simulink model "wlan_phy_tx_pmd"  (Simulink 7.8)
settings: Solver=ode45  StartTime=0.0  StopTime=Sim_Time  RelTol=1e-3
PostLoadFcn:
  | wlan_phy_tx_init
InitFcn:
  | wlan_phy_tx_init
StartFcn:
  | wlan_phy_tx_init
values from neighbouring files (symbols this model uses):
  interleave_64QAM_addr = interleave_64QAM + 2*floor(interleave_64QAM/6)    [wlan_phy_tx_init.m]
  MAX_NUM_BYTES = 4096    [wlan_phy_tx_init.m]
  MAX_NUM_SC = 64    [wlan_phy_tx_init.m]
  Preamble_IQ = PLCP_Preamble.Preamble_t    [wlan_phy_tx_init.m]
  Preamble_IQ_scaled = ALL_MOD_SCALING * Preamble_IQ    [wlan_phy_tx_init.m]
  Sim_Tx_Start_Period = 1*(160 * Tx_Time_usec) + 2e3    [wlan_phy_tx_init.m]
undefined symbols (not defined in the file or in its folder): gcbh, interleave_16QAM, interleave_bpsk, interleave_QPSK, Mod_Constellation_16QAM, Mod_Constellation_64QAM, Mod_Constellation_BPSK, Mod_Constellation_QPSK, xlBlockLoadCallback, xlGetNormalizedPeriod
libraries: xbsIndex_r4 x1173, xbsEDKLib_r4 x1
(part 5 of 8)

== system wlan_phy_tx_pmd/FIFO/I/Q Slice ==
  IQ : Inport
  Reinterpret2 : xbsIndex_r4/Reinterpret  force_arith_type=on  arith_type="Signed  (2's comp)"  force_bin_pt=on  bin_pt=15  block_type=reinterpret
  Reinterpret3 : xbsIndex_r4/Reinterpret  force_arith_type=on  arith_type="Signed  (2's comp)"  force_bin_pt=on  bin_pt=15  block_type=reinterpret
  Slice : xbsIndex_r4/Slice  nbits=16  boolean_output=off  mode=Upper Bit Location + Width  bit1=0  base1=MSB of Input  bit0=0  base0=LSB of Input  dbl_ovrd=off  block_type=slice
  Slice1 : xbsIndex_r4/Slice  nbits=16  boolean_output=off  mode=Lower Bit Location + Width  bit1=0  base1=MSB of Input  bit0=0  base0=LSB of Input  dbl_ovrd=off  block_type=slice
  I : Outport
  Q : Outport  Port=2
  wires:
  Reinterpret3/1 -> Q/1
  Reinterpret2/1 -> I/1
  IQ/1 -> Slice/1, Slice1/1
  Slice1/1 -> Reinterpret3/1
  Slice/1 -> Reinterpret2/1

== system wlan_phy_tx_pmd/Interleave & Modulate/16-QAM ==
  New Sym : Inport
  "bit tdata " : Inport  Port=2
  "bit tvalid " : Inport  Port=3
  data sym addr : Inport  Port=4
  16QAM Int Addr : Subsystem
  "16QAM Intlv " : Scope  NumInputPorts=7
      settings: TimeRange=15000  YMin=0~0~0~-0.1~0~0~-1  YMax=1~250~1~1.1~120~3~1  SaveName=ScopeData23
  Bit Memory1 : xbsIndex_r4/Dual Port RAM  depth=512  initVector=0  distributed_mem=Block RAM  init_a=0  init_b=0  rst_a=off  rst_b=off  en_a=off  en_b=off  latency=1  write_mode_A=Read After Write  write_mode_B=Read After Write  dbl_ovrd=off  optimize=Area  block_type=dpram
  Concat1 : xbsIndex_r4/Concat  num_inputs=2  dbl_ovrd=off  block_type=concat
  Concat2 : xbsIndex_r4/Concat  num_inputs=2  dbl_ovrd=off  block_type=concat
  Constant1 : xbsIndex_r4/Constant  const=0  gui_display_data_type=Fixed-point  arith_type=Unsigned  n_bits=4  bin_pt=0  preci_type=Single  exp_width=8  frac_width=24  explicit_period=off  period=1  equ=P=C  opselect=C  inp2=PCIN>>17  opr=+  inp1=P  carry=CIN  dbl_ovrd=off  block_type=constant
  Constant2 : xbsIndex_r4/Constant  const=0  gui_display_data_type=Boolean  arith_type=Boolean  n_bits=1  bin_pt=0  preci_type=Single  exp_width=8  frac_width=24  explicit_period=off  period=1  equ=P=C  opselect=C  inp2=PCIN>>17  opr=+  inp1=P  carry=CIN  dbl_ovrd=off  block_type=constant
  Delay2 : xbsIndex_r4/Delay  rst=off  infoeditControl=Selection of Reset will increase slice count due to use of real FFs and instead of SRLs  en=off  latency=1  dbl_ovrd=off  reg_retiming=off  block_type=delay
  Delay6 : xbsIndex_r4/Delay  rst=off  infoeditControl=Selection of Reset will increase slice count due to use of real FFs and instead of SRLs  en=off  latency=1  dbl_ovrd=off  reg_retiming=off  block_type=delay
  Gateway Out{1..5,8} (6 alike) : xbsIndex_r4/Gateway Out  inherit_from_input=off  hdl_port=off  timing_constraint=None  locs_specified=off  LOCs={}  UseAsDAC=off  DACChannel='1'  block_type=gatewayout
  Inverter : xbsIndex_r4/Inverter  en=off  latency=0  dbl_ovrd=off  block_type=inv
  Terminator : Terminator
  4b Data : Outport
  wires:
  Bit Memory1/2 -> 4b Data/1, Gateway Out5/1
  Bit Memory1/1 -> Terminator/1
  Inverter/1 -> Concat2/1
  data sym addr/1 -> Concat2/2
  Concat2/1 -> Bit Memory1/4, Gateway Out4/1
  Concat1/1 -> Bit Memory1/1, Gateway Out1/1
  16QAM Int Addr/2(Wr Addr) -> Concat1/2
  16QAM Int Addr/1(Wr Offset) -> Inverter/1, Concat1/1
  "bit tdata "/1 -> Delay6/1
  Constant2/1 -> Bit Memory1/6
  Constant1/1 -> Bit Memory1/5
  New Sym/1 -> 16QAM Int Addr/1(New Sym), Gateway Out8/1
  "bit tvalid "/1 -> 16QAM Int Addr/2(Bit Valid), Delay2/1
  Delay6/1 -> Bit Memory1/2, Gateway Out2/1
  Delay2/1 -> Bit Memory1/3, Gateway Out3/1
  Gateway Out8/1 -> "16QAM Intlv "/1  "New Sym"
  Gateway Out1/1 -> "16QAM Intlv "/2  "Wr Addr"
  Gateway Out2/1 -> "16QAM Intlv "/3  "Wr Bit"
  Gateway Out3/1 -> "16QAM Intlv "/4  "Wr En"
  Gateway Out4/1 -> "16QAM Intlv "/5  "Rd Addr"
  Gateway Out5/1 -> "16QAM Intlv "/6  "Rd Sym Out"

== system wlan_phy_tx_pmd/Interleave & Modulate/16QAM Mod ==
  note: 16-QAM Bit Mapping:
      | [b0 b1] / [b2 b3]:
      | 00 = -3
      | 01 = -1
      | 11 = +1
      | 10 = +3
      | Norm = 1/sqrt(10)
  note: 00 -> 00
  note: 10 -> 01
  note: 01 -> 10
  note: 11 -> 11
  b[3:0] : Inport
  Constant1 : xbsIndex_r4/Constant  const=Mod_Constellation_16QAM(3)  gui_display_data_type=Fixed-point  arith_type=Signed (2's comp)  n_bits=12  bin_pt=11  preci_type=Single  exp_width=8  frac_width=24  explicit_period=off  period=1  equ=P=C  opselect=C  inp2=PCIN>>17  opr=+  inp1=P  carry=CIN  dbl_ovrd=off  block_type=constant
  Constant2 : xbsIndex_r4/Constant  const=Mod_Constellation_16QAM(1)  gui_display_data_type=Fixed-point  arith_type=Signed (2's comp)  n_bits=12  bin_pt=11  preci_type=Single  exp_width=8  frac_width=24  explicit_period=off  period=1  equ=P=C  opselect=C  inp2=PCIN>>17  opr=+  inp1=P  carry=CIN  dbl_ovrd=off  block_type=constant
  Constant3 : xbsIndex_r4/Constant  const=Mod_Constellation_16QAM(2)  gui_display_data_type=Fixed-point  arith_type=Signed (2's comp)  n_bits=12  bin_pt=11  preci_type=Single  exp_width=8  frac_width=24  explicit_period=off  period=1  equ=P=C  opselect=C  inp2=PCIN>>17  opr=+  inp1=P  carry=CIN  dbl_ovrd=off  block_type=constant
  Constant4 : xbsIndex_r4/Constant  const=Mod_Constellation_16QAM(4)  gui_display_data_type=Fixed-point  arith_type=Signed (2's comp)  n_bits=12  bin_pt=11  preci_type=Single  exp_width=8  frac_width=24  explicit_period=off  period=1  equ=P=C  opselect=C  inp2=PCIN>>17  opr=+  inp1=P  carry=CIN  dbl_ovrd=off  block_type=constant
  Mux : xbsIndex_r4/Mux  inputs=4  en=off  latency=0  precision=Full  arith_type=Unsigned  n_bits=16  bin_pt=14  quantization=Truncate  overflow=Wrap  dbl_ovrd=off  block_type=mux
  Mux1 : xbsIndex_r4/Mux  inputs=4  en=off  latency=0  precision=Full  arith_type=Unsigned  n_bits=16  bin_pt=14  quantization=Truncate  overflow=Wrap  dbl_ovrd=off  block_type=mux
  b[1:0] : xbsIndex_r4/Slice  nbits=2  boolean_output=off  mode=Lower Bit Location + Width  bit1=0  base1=MSB of Input  bit0=0  base0=LSB of Input  dbl_ovrd=off  block_type=slice
  b[3:2] : xbsIndex_r4/Slice  nbits=2  boolean_output=off  mode=Lower Bit Location + Width  bit1=0  base1=MSB of Input  bit0=2  base0=LSB of Input  dbl_ovrd=off  block_type=slice
  I : Outport
  Q : Outport  Port=2
  wires:
  b[1:0]/1 -> Mux/1
  b[3:0]/1 -> b[1:0]/1, b[3:2]/1
  Constant2/1 -> Mux/2, Mux1/2
  Constant1/1 -> Mux/3, Mux1/3
  Constant3/1 -> Mux/4, Mux1/4
  Constant4/1 -> Mux/5, Mux1/5
  b[3:2]/1 -> Mux1/1
  Mux/1 -> I/1
  Mux1/1 -> Q/1

== system wlan_phy_tx_pmd/Interleave & Modulate/64-QAM ==
  New Sym : Inport
  "bit tdata " : Inport  Port=2
  "bit tvalid " : Inport  Port=3
  data sym addr : Inport  Port=4
  64QAM Int Addr : Subsystem
  "64QAM Intlv " : Scope  NumInputPorts=7
      settings: TimeRange=10000  YMin=0~0~0~-0.1~0~0~-1  YMax=1~250~1~1.1~120~3~1  SaveName=ScopeData23
  Bit Memory1 : xbsIndex_r4/Dual Port RAM  depth=1024  initVector=0  distributed_mem=Block RAM  init_a=0  init_b=0  rst_a=off  rst_b=off  en_a=off  en_b=off  latency=1  write_mode_A=Read After Write  write_mode_B=Read After Write  dbl_ovrd=off  optimize=Area  block_type=dpram
  Concat1 : xbsIndex_r4/Concat  num_inputs=2  dbl_ovrd=off  block_type=concat
  Concat2 : xbsIndex_r4/Concat  num_inputs=2  dbl_ovrd=off  block_type=concat
  Constant1 : xbsIndex_r4/Constant  const=0  gui_display_data_type=Fixed-point  arith_type=Unsigned  n_bits=8  bin_pt=0  preci_type=Single  exp_width=8  frac_width=24  explicit_period=off  period=1  equ=P=C  opselect=C  inp2=PCIN>>17  opr=+  inp1=P  carry=CIN  dbl_ovrd=off  block_type=constant
  Constant2 : xbsIndex_r4/Constant  const=0  gui_display_data_type=Boolean  arith_type=Boolean  n_bits=1  bin_pt=0  preci_type=Single  exp_width=8  frac_width=24  explicit_period=off  period=1  equ=P=C  opselect=C  inp2=PCIN>>17  opr=+  inp1=P  carry=CIN  dbl_ovrd=off  block_type=constant
  Delay2 : xbsIndex_r4/Delay  rst=off  infoeditControl=Selection of Reset will increase slice count due to use of real FFs and instead of SRLs  en=off  latency=1  dbl_ovrd=off  reg_retiming=off  block_type=delay
  Delay6 : xbsIndex_r4/Delay  rst=off  infoeditControl=Selection of Reset will increase slice count due to use of real FFs and instead of SRLs  en=off  latency=1  dbl_ovrd=off  reg_retiming=off  block_type=delay
  Gateway Out{1..6,8} (7 alike) : xbsIndex_r4/Gateway Out  inherit_from_input=off  hdl_port=off  timing_constraint=None  locs_specified=off  LOCs={}  UseAsDAC=off  DACChannel='1'  block_type=gatewayout
  Inverter : xbsIndex_r4/Inverter  en=off  latency=0  dbl_ovrd=off  block_type=inv
  Slice : xbsIndex_r4/Slice  nbits=6  boolean_output=off  mode=Lower Bit Location + Width  bit1=0  base1=MSB of Input  bit0=0  base0=LSB of Input  dbl_ovrd=off  block_type=slice
  Terminator : Terminator
  6b Data : Outport
  wires:
  Gateway Out5/1 -> "64QAM Intlv "/6  "Rd Sym Out"
  Gateway Out4/1 -> "64QAM Intlv "/5  "Rd Addr"
  Gateway Out3/1 -> "64QAM Intlv "/4  "Wr En"
  Gateway Out2/1 -> "64QAM Intlv "/3  "Wr Bit"
  Gateway Out1/1 -> "64QAM Intlv "/2  "Wr Addr"
  Gateway Out8/1 -> "64QAM Intlv "/1  "New Sym"
  Delay2/1 -> Gateway Out3/1, Bit Memory1/3
  Delay6/1 -> Gateway Out2/1, Bit Memory1/2
  "bit tvalid "/1 -> Delay2/1, 64QAM Int Addr/2(Bit Valid)
  New Sym/1 -> Gateway Out8/1, 64QAM Int Addr/1(New Sym)
  Constant1/1 -> Bit Memory1/5
  Constant2/1 -> Bit Memory1/6
  "bit tdata "/1 -> Delay6/1
  64QAM Int Addr/1(Wr Offset) -> Concat1/1, Inverter/1
  64QAM Int Addr/2(Wr Addr) -> Concat1/2
  Concat1/1 -> Gateway Out1/1, Bit Memory1/1
  Concat2/1 -> Gateway Out4/1, Bit Memory1/4
  data sym addr/1 -> Concat2/2
  Inverter/1 -> Concat2/1
  Bit Memory1/1 -> Terminator/1
  Bit Memory1/2 -> Gateway Out5/1, Slice/1
  Slice/1 -> 6b Data/1, Gateway Out6/1
  Gateway Out6/1 -> "64QAM Intlv "/7

== system wlan_phy_tx_pmd/Interleave & Modulate/64QAM Mod ==
  note: 64-QAM Bit Mapping:
      | [b0 b1 b2] / [b3 b4 b5]:
      | 000 = -7
      | 001 = -5
      | 010 = -1
      | 011 = -3
      | 100 = +7
      | 101 = +5
      | 110 = +1
      | 111 = +3
      |
      | Norm = 1/sqrt(42)
  note: Endian swap here - mux sel is [b2 b1 b0] / [b5 b4 b3]
  note: 000
  note: 001
  note: 010
  note: 011
  note: 100
  note: 101
  note: 110
  note: 111
  b[5:0] : Inport
  Constant1 : xbsIndex_r4/Constant  const=Mod_Constellation_64QAM(5)  gui_display_data_type=Fixed-point  arith_type=Signed (2's comp)  n_bits=12  bin_pt=11  preci_type=Single  exp_width=8  frac_width=24  explicit_period=off  period=1  equ=P=C  opselect=C  inp2=PCIN>>17  opr=+  inp1=P  carry=CIN  dbl_ovrd=off  block_type=constant
  Constant10 : xbsIndex_r4/Constant  const=Mod_Constellation_64QAM(2)  gui_display_data_type=Fixed-point  arith_type=Signed (2's comp)  n_bits=12  bin_pt=11  preci_type=Single  exp_width=8  frac_width=24  explicit_period=off  period=1  equ=P=C  opselect=C  inp2=PCIN>>17  opr=+  inp1=P  carry=CIN  dbl_ovrd=off  block_type=constant
  Constant11 : xbsIndex_r4/Constant  const=Mod_Constellation_64QAM(4)  gui_display_data_type=Fixed-point  arith_type=Signed (2's comp)  n_bits=12  bin_pt=11  preci_type=Single  exp_width=8  frac_width=24  explicit_period=off  period=1  equ=P=C  opselect=C  inp2=PCIN>>17  opr=+  inp1=P  carry=CIN  dbl_ovrd=off  block_type=constant
  Constant12 : xbsIndex_r4/Constant  const=Mod_Constellation_64QAM(8)  gui_display_data_type=Fixed-point  arith_type=Signed (2's comp)  n_bits=12  bin_pt=11  preci_type=Single  exp_width=8  frac_width=24  explicit_period=off  period=1  equ=P=C  opselect=C  inp2=PCIN>>17  opr=+  inp1=P  carry=CIN  dbl_ovrd=off  block_type=constant
  Constant13 : xbsIndex_r4/Constant  const=Mod_Constellation_64QAM(1)  gui_display_data_type=Fixed-point  arith_type=Signed (2's comp)  n_bits=12  bin_pt=11  preci_type=Single  exp_width=8  frac_width=24  explicit_period=off  period=1  equ=P=C  opselect=C  inp2=PCIN>>17  opr=+  inp1=P  carry=CIN  dbl_ovrd=off  block_type=constant
  Constant14 : xbsIndex_r4/Constant  const=Mod_Constellation_64QAM(3)  gui_display_data_type=Fixed-point  arith_type=Signed (2's comp)  n_bits=12  bin_pt=11  preci_type=Single  exp_width=8  frac_width=24  explicit_period=off  period=1  equ=P=C  opselect=C  inp2=PCIN>>17  opr=+  inp1=P  carry=CIN  dbl_ovrd=off  block_type=constant
  Constant15 : xbsIndex_r4/Constant  const=Mod_Constellation_64QAM(7)  gui_display_data_type=Fixed-point  arith_type=Signed (2's comp)  n_bits=12  bin_pt=11  preci_type=Single  exp_width=8  frac_width=24  explicit_period=off  period=1  equ=P=C  opselect=C  inp2=PCIN>>17  opr=+  inp1=P  carry=CIN  dbl_ovrd=off  block_type=constant
  Constant16 : xbsIndex_r4/Constant  const=Mod_Constellation_64QAM(6)  gui_display_data_type=Fixed-point  arith_type=Signed (2's comp)  n_bits=12  bin_pt=11  preci_type=Single  exp_width=8  frac_width=24  explicit_period=off  period=1  equ=P=C  opselect=C  inp2=PCIN>>17  opr=+  inp1=P  carry=CIN  dbl_ovrd=off  block_type=constant
  Constant2 : xbsIndex_r4/Constant  const=Mod_Constellation_64QAM(1)  gui_display_data_type=Fixed-point  arith_type=Signed (2's comp)  n_bits=12  bin_pt=11  preci_type=Single  exp_width=8  frac_width=24  explicit_period=off  period=1  equ=P=C  opselect=C  inp2=PCIN>>17  opr=+  inp1=P  carry=CIN  dbl_ovrd=off  block_type=constant
  Constant3 : xbsIndex_r4/Constant  const=Mod_Constellation_64QAM(3)  gui_display_data_type=Fixed-point  arith_type=Signed (2's comp)  n_bits=12  bin_pt=11  preci_type=Single  exp_width=8  frac_width=24  explicit_period=off  period=1  equ=P=C  opselect=C  inp2=PCIN>>17  opr=+  inp1=P  carry=CIN  dbl_ovrd=off  block_type=constant
  Constant4 : xbsIndex_r4/Constant  const=Mod_Constellation_64QAM(7)  gui_display_data_type=Fixed-point  arith_type=Signed (2's comp)  n_bits=12  bin_pt=11  preci_type=Single  exp_width=8  frac_width=24  explicit_period=off  period=1  equ=P=C  opselect=C  inp2=PCIN>>17  opr=+  inp1=P  carry=CIN  dbl_ovrd=off  block_type=constant
  Constant5 : xbsIndex_r4/Constant  const=Mod_Constellation_64QAM(5)  gui_display_data_type=Fixed-point  arith_type=Signed (2's comp)  n_bits=12  bin_pt=11  preci_type=Single  exp_width=8  frac_width=24  explicit_period=off  period=1  equ=P=C  opselect=C  inp2=PCIN>>17  opr=+  inp1=P  carry=CIN  dbl_ovrd=off  block_type=constant
  Constant6 : xbsIndex_r4/Constant  const=Mod_Constellation_64QAM(2)  gui_display_data_type=Fixed-point  arith_type=Signed (2's comp)  n_bits=12  bin_pt=11  preci_type=Single  exp_width=8  frac_width=24  explicit_period=off  period=1  equ=P=C  opselect=C  inp2=PCIN>>17  opr=+  inp1=P  carry=CIN  dbl_ovrd=off  block_type=constant
  Constant7 : xbsIndex_r4/Constant  const=Mod_Constellation_64QAM(4)  gui_display_data_type=Fixed-point  arith_type=Signed (2's comp)  n_bits=12  bin_pt=11  preci_type=Single  exp_width=8  frac_width=24  explicit_period=off  period=1  equ=P=C  opselect=C  inp2=PCIN>>17  opr=+  inp1=P  carry=CIN  dbl_ovrd=off  block_type=constant
  Constant8 : xbsIndex_r4/Constant  const=Mod_Constellation_64QAM(8)  gui_display_data_type=Fixed-point  arith_type=Signed (2's comp)  n_bits=12  bin_pt=11  preci_type=Single  exp_width=8  frac_width=24  explicit_period=off  period=1  equ=P=C  opselect=C  inp2=PCIN>>17  opr=+  inp1=P  carry=CIN  dbl_ovrd=off  block_type=constant
  Constant9 : xbsIndex_r4/Constant  const=Mod_Constellation_64QAM(6)  gui_display_data_type=Fixed-point  arith_type=Signed (2's comp)  n_bits=12  bin_pt=11  preci_type=Single  exp_width=8  frac_width=24  explicit_period=off  period=1  equ=P=C  opselect=C  inp2=PCIN>>17  opr=+  inp1=P  carry=CIN  dbl_ovrd=off  block_type=constant
  Mux : xbsIndex_r4/Mux  inputs=8  en=off  latency=0  precision=Full  arith_type=Unsigned  n_bits=16  bin_pt=14  quantization=Truncate  overflow=Wrap  dbl_ovrd=off  block_type=mux
  Mux1 : xbsIndex_r4/Mux  inputs=8  en=off  latency=0  precision=Full  arith_type=Unsigned  n_bits=16  bin_pt=14  quantization=Truncate  overflow=Wrap  dbl_ovrd=off  block_type=mux
  b[2:0] : xbsIndex_r4/Slice  nbits=3  boolean_output=off  mode=Lower Bit Location + Width  bit1=0  base1=MSB of Input  bit0=0  base0=LSB of Input  dbl_ovrd=off  block_type=slice
  b[5:3] : xbsIndex_r4/Slice  nbits=3  boolean_output=off  mode=Lower Bit Location + Width  bit1=0  base1=MSB of Input  bit0=3  base0=LSB of Input  dbl_ovrd=off  block_type=slice
  I : Outport
  Q : Outport  Port=2
  wires:
  Constant4/1 -> Mux/5
  Constant3/1 -> Mux/4
  Constant1/1 -> Mux/3
  Constant2/1 -> Mux/2
  b[5:0]/1 -> b[5:3]/1, b[2:0]/1
  b[2:0]/1 -> Mux/1
  Constant10/1 -> Mux/6
  Constant9/1 -> Mux/7
  Constant11/1 -> Mux/8
  Constant12/1 -> Mux/9
  Mux/1 -> I/1
  Constant15/1 -> Mux1/5
  Constant14/1 -> Mux1/4
  Constant5/1 -> Mux1/3
  Constant13/1 -> Mux1/2
  Constant6/1 -> Mux1/6
  Constant16/1 -> Mux1/7
  Constant7/1 -> Mux1/8
  Constant8/1 -> Mux1/9
  b[5:3]/1 -> Mux1/1
  Mux1/1 -> Q/1

== system wlan_phy_tx_pmd/Interleave & Modulate/BPSK ==
  New Sym : Inport
  "bit tdata " : Inport  Port=2
  "bit tvalid " : Inport  Port=3
  data sym addr : Inport  Port=4
  BPSK Int Addr : Subsystem
  "BSPK Intlv " : Scope  NumInputPorts=7
      settings: TimeRange=10000  YMin=0~0~-0.1~-2~0~-0.1~-0.1  YMax=300~300~1.1~2~4000~1.1~1.1  SaveName=ScopeData15
  Bit Memory : xbsIndex_r4/Dual Port RAM  depth=128  initVector=0  distributed_mem=Block RAM  init_a=0  init_b=0  rst_a=off  rst_b=off  en_a=off  en_b=off  latency=1  write_mode_A=Read After Write  write_mode_B=Read After Write  dbl_ovrd=off  optimize=Area  block_type=dpram
  Concat1 : xbsIndex_r4/Concat  num_inputs=2  dbl_ovrd=off  block_type=concat
  Concat2 : xbsIndex_r4/Concat  num_inputs=2  dbl_ovrd=off  block_type=concat
  Constant1 : xbsIndex_r4/Constant  const=0  gui_display_data_type=Fixed-point  arith_type=Unsigned  n_bits=1  bin_pt=0  preci_type=Single  exp_width=8  frac_width=24  explicit_period=off  period=1  equ=P=C  opselect=C  inp2=PCIN>>17  opr=+  inp1=P  carry=CIN  dbl_ovrd=off  block_type=constant
  Constant2 : xbsIndex_r4/Constant  const=0  gui_display_data_type=Boolean  arith_type=Boolean  n_bits=1  bin_pt=0  preci_type=Single  exp_width=8  frac_width=24  explicit_period=off  period=1  equ=P=C  opselect=C  inp2=PCIN>>17  opr=+  inp1=P  carry=CIN  dbl_ovrd=off  block_type=constant
  Delay1 : xbsIndex_r4/Delay  rst=off  infoeditControl=Selection of Reset will increase slice count due to use of real FFs and instead of SRLs  en=off  latency=1  dbl_ovrd=off  reg_retiming=off  block_type=delay
  Delay6 : xbsIndex_r4/Delay  rst=off  infoeditControl=Selection of Reset will increase slice count due to use of real FFs and instead of SRLs  en=off  latency=1  dbl_ovrd=off  reg_retiming=off  block_type=delay
  Gateway Out{1..5,8} (6 alike) : xbsIndex_r4/Gateway Out  inherit_from_input=off  hdl_port=off  timing_constraint=None  locs_specified=off  LOCs={}  UseAsDAC=off  DACChannel='1'  block_type=gatewayout
  Inverter : xbsIndex_r4/Inverter  en=off  latency=0  dbl_ovrd=off  block_type=inv
  Terminator : Terminator
  1b Data : Outport
  wires:
  "bit tvalid "/1 -> BPSK Int Addr/2(Bit Valid), Delay1/1
  New Sym/1 -> BPSK Int Addr/1(New Sym), Gateway Out8/1
  Constant1/1 -> Bit Memory/5
  Constant2/1 -> Bit Memory/6
  "bit tdata "/1 -> Delay6/1
  BPSK Int Addr/1(Wr Offset) -> Concat1/1, Inverter/1
  BPSK Int Addr/2(Wr Addr) -> Concat1/2
  Concat1/1 -> Bit Memory/1, Gateway Out1/1
  Concat2/1 -> Bit Memory/4, Gateway Out4/1
  data sym addr/1 -> Concat2/2
  Inverter/1 -> Concat2/1
  Bit Memory/1 -> Terminator/1
  Bit Memory/2 -> 1b Data/1, Gateway Out5/1
  Gateway Out8/1 -> "BSPK Intlv "/1
  Gateway Out1/1 -> "BSPK Intlv "/2
  Gateway Out2/1 -> "BSPK Intlv "/3
  Gateway Out3/1 -> "BSPK Intlv "/4
  Gateway Out4/1 -> "BSPK Intlv "/5
  Gateway Out5/1 -> "BSPK Intlv "/6
  Delay6/1 -> Bit Memory/2, Gateway Out2/1
  Delay1/1 -> Bit Memory/3, Gateway Out3/1

== system wlan_phy_tx_pmd/Interleave & Modulate/BPSK Mod ==
  b[0] : Inport
  Constant2 : xbsIndex_r4/Constant  const=Mod_Constellation_BPSK(1)  gui_display_data_type=Fixed-point  arith_type=Signed (2's comp)  n_bits=12  bin_pt=11  preci_type=Single  exp_width=8  frac_width=24  explicit_period=off  period=1  equ=P=C  opselect=C  inp2=PCIN>>17  opr=+  inp1=P  carry=CIN  dbl_ovrd=off  block_type=constant
  Constant3 : xbsIndex_r4/Constant  const=Mod_Constellation_BPSK(2)  gui_display_data_type=Fixed-point  arith_type=Signed (2's comp)  n_bits=12  bin_pt=11  preci_type=Single  exp_width=8  frac_width=24  explicit_period=off  period=1  equ=P=C  opselect=C  inp2=PCIN>>17  opr=+  inp1=P  carry=CIN  dbl_ovrd=off  block_type=constant
  Constant4 : xbsIndex_r4/Constant  const=0  gui_display_data_type=Fixed-point  arith_type=Signed (2's comp)  n_bits=12  bin_pt=11  preci_type=Single  exp_width=8  frac_width=24  explicit_period=off  period=1  equ=P=C  opselect=C  inp2=PCIN>>17  opr=+  inp1=P  carry=CIN  dbl_ovrd=off  block_type=constant
  Mux : xbsIndex_r4/Mux  inputs=2  en=off  latency=0  precision=Full  arith_type=Unsigned  n_bits=16  bin_pt=14  quantization=Truncate  overflow=Wrap  dbl_ovrd=off  block_type=mux
  I : Outport
  Q : Outport  Port=2
  wires:
  Mux/1 -> I/1
  Constant3/1 -> Mux/3
  Constant2/1 -> Mux/2
  b[0]/1 -> Mux/1
  Constant4/1 -> Q/1

== system wlan_phy_tx_pmd/Interleave & Modulate/Coded Bit Counter ==
  Bit valid : Inport
  Constant3 : xbsIndex_r4/Constant  const=48  gui_display_data_type=Fixed-point  arith_type=Unsigned  n_bits=6  bin_pt=0  preci_type=Single  exp_width=8  frac_width=24  explicit_period=off  period=1  equ=P=C  opselect=C  inp2=PCIN>>17  opr=+  inp1=P  carry=CIN  dbl_ovrd=off  block_type=constant
  Delay2 : xbsIndex_r4/Delay  rst=off  infoeditControl=Selection of Reset will increase slice count due to use of real FFs and instead of SRLs  en=off  latency=1  dbl_ovrd=off  reg_retiming=off  block_type=delay
  Gateway Out{1..4,8} (5 alike) : xbsIndex_r4/Gateway Out  inherit_from_input=off  hdl_port=off  timing_constraint=None  locs_specified=off  LOCs={}  UseAsDAC=off  DACChannel='1'  block_type=gatewayout
  Inverter : xbsIndex_r4/Inverter  en=off  latency=0  dbl_ovrd=off  block_type=inv
      settings: xl_area=[0 0 0 0 0 0 0]  block_version=VER_STRING_GOES_HERE
  Logical1 : xbsIndex_r4/Logical  logical_function=OR  inputs=2  en=off  latency=0  precision=Full  arith_type=Unsigned  n_bits=8  bin_pt=2  align_bp=on  dbl_ovrd=off  block_type=logical
      settings: xl_area=[1 0 0 1 0 0 0]  block_version=VER_STRING_GOES_HERE
  Logical2 : xbsIndex_r4/Logical  logical_function=AND  inputs=2  en=off  latency=0  precision=Full  arith_type=Unsigned  n_bits=8  bin_pt=2  align_bp=on  dbl_ovrd=off  block_type=logical
      settings: xl_area=[1 0 0 1 0 0 0]  block_version=VER_STRING_GOES_HERE
  Mux : xbsIndex_r4/Mux  inputs=2  en=off  latency=0  precision=Full  arith_type=Unsigned  n_bits=16  bin_pt=14  quantization=Truncate  overflow=Wrap  dbl_ovrd=off  block_type=mux
  Relational2 : xbsIndex_r4/Relational  mode=a<b  en=off  latency=0  dbl_ovrd=off  block_type=relational
  S-R Latch2 : Subsystem
  Sym Coded Bit Count : xbsIndex_r4/Counter  cnt_type=Free Running  cnt_to=Inf  operation=Up  start_count=1  cnt_by_val=1  arith_type=Unsigned  n_bits=9  bin_pt=0  load_pin=off  rst=on  en=on  explicit_period=off  period=1  dbl_ovrd=off  use_behavioral_HDL=off  implementation=Fabric  block_type=counter
  Sym Coded Bit Count1 : Scope  NumInputPorts=7
      settings: TimeRange=15000  YMin=0~0~0~0~0~-1~-1  YMax=1~100~1~1~1~1~1  SaveName=ScopeData5
  Bits Ready : Outport
  wires:
  [DATA_N_CBPS] -> Mux/3
  Constant3/1 -> Mux/2
  Mux/1 -> Relational2/2
  Sym Coded Bit Count/1 -> Gateway Out1/1, Relational2/1
  Logical1/1 -> Sym Coded Bit Count/1
  S-R Latch2/1(Q) -> Mux/1, Gateway Out4/1
  Bit valid/1 -> Sym Coded Bit Count/2, Gateway Out8/1, Logical2/2
  Logical2/1 -> Logical1/1, S-R Latch2/1(S), Gateway Out3/1, Delay2/1
  [TX_RESET] -> S-R Latch2/2(R), Logical1/2
  Gateway Out8/1 -> Sym Coded Bit Count1/1
  Gateway Out1/1 -> Sym Coded Bit Count1/2
  Gateway Out2/1 -> Sym Coded Bit Count1/3
  Gateway Out3/1 -> Sym Coded Bit Count1/4
  Gateway Out4/1 -> Sym Coded Bit Count1/5
  Delay2/1 -> Bits Ready/1
  Relational2/1 -> Inverter/1
  Inverter/1 -> Logical2/1, Gateway Out2/1

== system wlan_phy_tx_pmd/Interleave & Modulate/Control & Pilots ==
  note: SC Counter EN high extra cycle post wrap reset
      | (due to SR latch latency?)
  note: 1 cycle for RAM access
  note: May need tweaked delay to handle edge
      | case of 1 required bit alone in final
      | symbol
  Bits Ready : Inport
  FIFO Ready : Inport  Port=2
  Concat1 : xbsIndex_r4/Concat  num_inputs=2  dbl_ovrd=off  block_type=concat
  Data SC Map : Subsystem
  Delay{,1..3,5..6} (6 alike) : xbsIndex_r4/Delay  rst=off  infoeditControl=Selection of Reset will increase slice count due to use of real FFs and instead of SRLs  en=off  latency=1  dbl_ovrd=off  reg_retiming=off  block_type=delay
  Delay4 : xbsIndex_r4/Delay  rst=off  infoeditControl=Selection of Reset will increase slice count due to use of real FFs and instead of SRLs  en=off  latency=0  dbl_ovrd=off  reg_retiming=off  block_type=delay
  Gateway Out{1..4,8} (5 alike) : xbsIndex_r4/Gateway Out  inherit_from_input=off  hdl_port=off  timing_constraint=None  locs_specified=off  LOCs={}  UseAsDAC=off  DACChannel='1'  block_type=gatewayout
  Logical : xbsIndex_r4/Logical  logical_function=OR  inputs=2  en=off  latency=0  precision=Full  arith_type=Unsigned  n_bits=8  bin_pt=2  align_bp=on  dbl_ovrd=off  block_type=logical
      settings: xl_area=[0, 0, 0, 0, 0, 0, 0]  block_version=VER_STRING_GOES_HERE
  Logical1 : xbsIndex_r4/Logical  logical_function=AND  inputs=2  en=off  latency=0  precision=Full  arith_type=Unsigned  n_bits=8  bin_pt=2  align_bp=on  dbl_ovrd=off  block_type=logical
      settings: xl_area=[0, 0, 0, 0, 0, 0, 0]  block_version=VER_STRING_GOES_HERE
  Logical2 : xbsIndex_r4/Logical  logical_function=AND  inputs=2  en=off  latency=0  precision=Full  arith_type=Unsigned  n_bits=8  bin_pt=2  align_bp=on  dbl_ovrd=off  block_type=logical
      settings: xl_area=[0, 0, 0, 0, 0, 0, 0]  block_version=VER_STRING_GOES_HERE
  Mod Ctrl : Scope  NumInputPorts=7
      settings: TimeRange=10000  YMin=0~0~0~-0.1~0~-0.1~-0.1  YMax=300~300~1~1.1~4000~1.1~1.1  SaveName=ScopeData4
  Pilot Gen : Subsystem
  Posedge : Subsystem
  Posedge1 : Subsystem
  S-R Latch1 : Subsystem
  S-R Latch2 : Subsystem
  Subcarrier Index Count : Subsystem
  data sym ind : Outport
  DATA : Outport  Port=2
  Pilot I : Outport  Port=3
  IQ Sel : Outport  Port=4
  Last Samp : Outport  Port=5
  IQ Valid : Outport  Port=6
  " Last Sym" : Outport  Port=7
  wires:
  Subcarrier Index Count/1(sc_ind) -> Data SC Map/1(sc_ind), Pilot Gen/1(sc_ind)
  Pilot Gen/1(pilot_valid) -> Concat1/2
  Data SC Map/2(data_sym_valid) -> Concat1/1
  Data SC Map/1(data_sym_ind) -> data sym ind/1
  Concat1/1 -> Delay5/1
  Pilot Gen/2(Pilot_I) -> Delay6/1
  [TX_RESET] -> Subcarrier Index Count/2(reset), Pilot Gen/2(reset), Logical/1, S-R Latch2/2(R)
  Bits Ready/1 -> Posedge/1(D), Gateway Out8/1
  Posedge/1(Q) -> S-R Latch1/1(S)
  Subcarrier Index Count/2(last) -> Logical/2, Delay1/1, S-R Latch2/1(S), Logical2/1
  Posedge1/1(Q) -> S-R Latch1/2(R)
  Logical/1 -> Posedge1/1(D)
  Logical1/1 -> Subcarrier Index Count/1(en)
  FIFO Ready/1 -> Logical1/2
  S-R Latch1/1(Q) -> Logical1/1, Delay/1
  S-R Latch2/1(Q) -> Delay2/1
  Delay/1 -> IQ Valid/1, Gateway Out1/1
  Delay1/1 -> Last Samp/1, Gateway Out2/1
  Delay2/1 -> DATA/1, Gateway Out3/1
  Gateway Out8/1 -> Mod Ctrl/1
  Gateway Out1/1 -> Mod Ctrl/2
  Gateway Out2/1 -> Mod Ctrl/3
  Gateway Out3/1 -> Mod Ctrl/4
  Delay3/1 -> " Last Sym"/1, Gateway Out4/1
  [PPDU_TAIL_DONE] -> Delay4/1
  Logical2/1 -> Delay3/1
  Gateway Out4/1 -> Mod Ctrl/5
  Delay4/1 -> Logical2/2
  Delay5/1 -> IQ Sel/1
  Delay6/1 -> Pilot I/1

== system wlan_phy_tx_pmd/Interleave & Modulate/QPSK ==
  New Sym : Inport
  "bit tdata " : Inport  Port=2
  "bit tvalid " : Inport  Port=3
  data sym addr : Inport  Port=4
  Bit Memory1 : xbsIndex_r4/Dual Port RAM  depth=256  initVector=0  distributed_mem=Block RAM  init_a=0  init_b=0  rst_a=off  rst_b=off  en_a=off  en_b=off  latency=1  write_mode_A=Read After Write  write_mode_B=Read After Write  dbl_ovrd=off  optimize=Area  block_type=dpram
  Concat1 : xbsIndex_r4/Concat  num_inputs=2  dbl_ovrd=off  block_type=concat
  Concat2 : xbsIndex_r4/Concat  num_inputs=2  dbl_ovrd=off  block_type=concat
  Constant1 : xbsIndex_r4/Constant  const=0  gui_display_data_type=Fixed-point  arith_type=Unsigned  n_bits=2  bin_pt=0  preci_type=Single  exp_width=8  frac_width=24  explicit_period=off  period=1  equ=P=C  opselect=C  inp2=PCIN>>17  opr=+  inp1=P  carry=CIN  dbl_ovrd=off  block_type=constant
  Constant2 : xbsIndex_r4/Constant  const=0  gui_display_data_type=Boolean  arith_type=Boolean  n_bits=1  bin_pt=0  preci_type=Single  exp_width=8  frac_width=24  explicit_period=off  period=1  equ=P=C  opselect=C  inp2=PCIN>>17  opr=+  inp1=P  carry=CIN  dbl_ovrd=off  block_type=constant
  Delay2 : xbsIndex_r4/Delay  rst=off  infoeditControl=Selection of Reset will increase slice count due to use of real FFs and instead of SRLs  en=off  latency=1  dbl_ovrd=off  reg_retiming=off  block_type=delay
  Delay6 : xbsIndex_r4/Delay  rst=off  infoeditControl=Selection of Reset will increase slice count due to use of real FFs and instead of SRLs  en=off  latency=1  dbl_ovrd=off  reg_retiming=off  block_type=delay
  Gateway Out{1..5,8} (6 alike) : xbsIndex_r4/Gateway Out  inherit_from_input=off  hdl_port=off  timing_constraint=None  locs_specified=off  LOCs={}  UseAsDAC=off  DACChannel='1'  block_type=gatewayout
  Inverter : xbsIndex_r4/Inverter  en=off  latency=0  dbl_ovrd=off  block_type=inv
  QPSK Int Addr : Subsystem
  "QSPK Intlv " : Scope  NumInputPorts=7
      settings: TimeRange=15000  YMin=0~0~0~-0.1~0~0~-1  YMax=1~250~1~1.1~120~3~1  SaveName=ScopeData16
  Terminator : Terminator
  2b Data : Outport
  wires:
  Bit Memory1/2 -> 2b Data/1, Gateway Out5/1
  Bit Memory1/1 -> Terminator/1
  Inverter/1 -> Concat2/1
  data sym addr/1 -> Concat2/2
  Concat2/1 -> Bit Memory1/4, Gateway Out4/1
  Concat1/1 -> Bit Memory1/1, Gateway Out1/1
  QPSK Int Addr/2(Wr Addr) -> Concat1/2
  QPSK Int Addr/1(Wr Offset) -> Inverter/1, Concat1/1
  "bit tdata "/1 -> Delay6/1
  Constant2/1 -> Bit Memory1/6
  Constant1/1 -> Bit Memory1/5
  New Sym/1 -> QPSK Int Addr/1(New Sym), Gateway Out8/1
  "bit tvalid "/1 -> QPSK Int Addr/2(Bit Valid), Delay2/1
  Delay6/1 -> Bit Memory1/2, Gateway Out2/1
  Delay2/1 -> Bit Memory1/3, Gateway Out3/1
  Gateway Out8/1 -> "QSPK Intlv "/1  "New Sym"
  Gateway Out1/1 -> "QSPK Intlv "/2  "Wr Addr"
  Gateway Out2/1 -> "QSPK Intlv "/3  "Wr Bit"
  Gateway Out3/1 -> "QSPK Intlv "/4  "Wr En"
  Gateway Out4/1 -> "QSPK Intlv "/5  "Rd Addr"
  Gateway Out5/1 -> "QSPK Intlv "/6  "Rd Sym Out"

== system wlan_phy_tx_pmd/Interleave & Modulate/QPSK Mod ==
  b[1:0] : Inport
  Constant2 : xbsIndex_r4/Constant  const=Mod_Constellation_QPSK(1)  gui_display_data_type=Fixed-point  arith_type=Signed (2's comp)  n_bits=12  bin_pt=11  preci_type=Single  exp_width=8  frac_width=24  explicit_period=off  period=1  equ=P=C  opselect=C  inp2=PCIN>>17  opr=+  inp1=P  carry=CIN  dbl_ovrd=off  block_type=constant
  Constant3 : xbsIndex_r4/Constant  const=Mod_Constellation_QPSK(2)  gui_display_data_type=Fixed-point  arith_type=Signed (2's comp)  n_bits=12  bin_pt=11  preci_type=Single  exp_width=8  frac_width=24  explicit_period=off  period=1  equ=P=C  opselect=C  inp2=PCIN>>17  opr=+  inp1=P  carry=CIN  dbl_ovrd=off  block_type=constant
  LSB : xbsIndex_r4/Slice  nbits=1  boolean_output=off  mode=Lower Bit Location + Width  bit1=0  base1=MSB of Input  bit0=0  base0=LSB of Input  dbl_ovrd=off  block_type=slice
  LSB+1 : xbsIndex_r4/Slice  nbits=1  boolean_output=off  mode=Lower Bit Location + Width  bit1=0  base1=MSB of Input  bit0=1  base0=LSB of Input  dbl_ovrd=off  block_type=slice
  Mux : xbsIndex_r4/Mux  inputs=2  en=off  latency=0  precision=Full  arith_type=Unsigned  n_bits=16  bin_pt=14  quantization=Truncate  overflow=Wrap  dbl_ovrd=off  block_type=mux
  Mux1 : xbsIndex_r4/Mux  inputs=2  en=off  latency=0  precision=Full  arith_type=Unsigned  n_bits=16  bin_pt=14  quantization=Truncate  overflow=Wrap  dbl_ovrd=off  block_type=mux
  I : Outport
  Q : Outport  Port=2
  wires:
  Mux1/1 -> Q/1
  Mux/1 -> I/1
  Constant3/1 -> Mux1/3, Mux/3
  Constant2/1 -> Mux1/2, Mux/2
  b[1:0]/1 -> LSB/1, LSB+1/1
  LSB/1 -> Mux/1
  LSB+1/1 -> Mux1/1

== system wlan_phy_tx_pmd/Preamble & Outputs/DAC Outputs ==
  En : Inport
  I : Inport  Port=2
  Q : Inport  Port=3
  Ant Enables : Subsystem
  Inverter{1..4} (4 alike) : xbsIndex_r4/Inverter  en=off  latency=0  dbl_ovrd=off  block_type=inv
      settings: xl_area=[0 0 0 0 0 0 0]  block_version=VER_STRING_GOES_HERE
  Logical{,1..3} (4 alike) : xbsIndex_r4/Logical  logical_function=AND  inputs=2  en=off  latency=0  precision=Full  arith_type=Unsigned  n_bits=16  bin_pt=0  align_bp=on  dbl_ovrd=off  block_type=logical
  RFA DAC I : xbsIndex_r4/Gateway Out  inherit_from_input=off  hdl_port=on  timing_constraint=None  locs_specified=off  LOCs={}  UseAsDAC=off  DACChannel='1'  block_type=gatewayout
  RFA DAC Q : xbsIndex_r4/Gateway Out  inherit_from_input=off  hdl_port=on  timing_constraint=None  locs_specified=off  LOCs={}  UseAsDAC=off  DACChannel='1'  block_type=gatewayout
  RFB DAC I : xbsIndex_r4/Gateway Out  inherit_from_input=off  hdl_port=on  timing_constraint=None  locs_specified=off  LOCs={}  UseAsDAC=off  DACChannel='1'  block_type=gatewayout
  RFB DAC Q : xbsIndex_r4/Gateway Out  inherit_from_input=off  hdl_port=on  timing_constraint=None  locs_specified=off  LOCs={}  UseAsDAC=off  DACChannel='1'  block_type=gatewayout
  RFC DAC I : xbsIndex_r4/Gateway Out  inherit_from_input=off  hdl_port=on  timing_constraint=None  locs_specified=off  LOCs={}  UseAsDAC=off  DACChannel='1'  block_type=gatewayout
  RFC DAC Q : xbsIndex_r4/Gateway Out  inherit_from_input=off  hdl_port=on  timing_constraint=None  locs_specified=off  LOCs={}  UseAsDAC=off  DACChannel='1'  block_type=gatewayout
  RFD DAC I : xbsIndex_r4/Gateway Out  inherit_from_input=off  hdl_port=on  timing_constraint=None  locs_specified=off  LOCs={}  UseAsDAC=off  DACChannel='1'  block_type=gatewayout
  RFD DAC Q : xbsIndex_r4/Gateway Out  inherit_from_input=off  hdl_port=on  timing_constraint=None  locs_specified=off  LOCs={}  UseAsDAC=off  DACChannel='1'  block_type=gatewayout
  Register{,1..7} (8 alike) : xbsIndex_r4/Register  init=0  rst=on  en=off  dbl_ovrd=off  block_type=register
  Register10 : xbsIndex_r4/Register  init=0  rst=off  en=off  dbl_ovrd=off  block_type=register
  Register8 : xbsIndex_r4/Register  init=0  rst=off  en=off  dbl_ovrd=off  block_type=register
  Register9 : xbsIndex_r4/Register  init=0  rst=off  en=off  dbl_ovrd=off  block_type=register
  " I" : Outport
  " Q" : Outport  Port=2
  wires:
  Register1/1 -> RFA DAC Q/1
  Register/1 -> RFA DAC I/1
  Inverter1/1 -> Register/2, Register1/2
  Logical/1 -> Inverter1/1
  I/1 -> Register8/1
  RFA DAC I/1 -> " I"/1
  Q/1 -> Register10/1
  RFA DAC Q/1 -> " Q"/1
  Register3/1 -> RFB DAC Q/1
  Register2/1 -> RFB DAC I/1
  En/1 -> Register9/1
  Ant Enables/1(A En) -> Logical/2
  Logical1/1 -> Inverter2/1
  Inverter2/1 -> Register2/2, Register3/2
  Ant Enables/2(B En) -> Logical1/2
  Register5/1 -> RFC DAC Q/1
  Register4/1 -> RFC DAC I/1
  Logical2/1 -> Inverter3/1
  Inverter3/1 -> Register5/2, Register4/2
  Register7/1 -> RFD DAC Q/1
  Register6/1 -> RFD DAC I/1
  Logical3/1 -> Inverter4/1
  Inverter4/1 -> Register6/2, Register7/2
  Ant Enables/4(D En) -> Logical3/2
  Register8/1 -> Register/1, Register2/1, Register4/1, Register6/1
  Register9/1 -> Logical/1, Logical1/1, Logical2/1, Logical3/1
  Register10/1 -> Register1/1, Register3/1, Register5/1, Register7/1
  Ant Enables/3(C En) -> Logical2/2

== system wlan_phy_tx_pmd/Preamble & Outputs/FIFO ==
  Reset : Inport
  FFT I : Inport  Port=2
  FFT Q : Inport  Port=3
  Write : Inport  Port=4
  Rd : Inport  Port=5
  Convert2 : xbsIndex_r4/Convert  gui_display_data_type=Boolean  arith_type=Boolean  n_bits=1  bin_pt=0  float_type=Single  exp_bits=8  fraction_bits=24  quantization=Truncate  overflow=Wrap  en=off  latency=0  dbl_ovrd=off  pipeline=off  block_type=convert
  Delay1 : xbsIndex_r4/Delay  rst=off  infoeditControl=Selection of Reset will increase slice count due to use of real FFs and instead of SRLs  en=off  latency=12  dbl_ovrd=off  reg_retiming=off  block_type=delay
  FIFO : xbsIndex_r4/FIFO  mem_type=Block RAM  performance_options=Standard_FIFO  infoedit1=Available only for V4, V5, V6, V7, K7, A7 and Zynq devices.  embedded_registers=on  depth=256  percent_nbits=1  rst=on  en=off  use_dcount=on  use_percent_full_port=off  use_almost_empty=off  almost_empty_thresh=2  use_almost_full=off  almost_full_thresh=14  dbl_ovrd=off  explicit_period=off  block_type=fifo
  I/Q Concat : Subsystem
  I/Q Slice : Subsystem
  Logical4 : xbsIndex_r4/Logical  logical_function=OR  inputs=2  en=off  latency=0  precision=Full  arith_type=Unsigned  n_bits=16  bin_pt=0  align_bp=on  dbl_ovrd=off  block_type=logical
  " I" : Outport
  " Q" : Outport  Port=2
  " Occ" : Outport  Port=3
  wires:
  FFT Q/1 -> I/Q Concat/2(Q)
  FFT I/1 -> I/Q Concat/1(I)
  I/Q Slice/2(Q) -> " Q"/1
  I/Q Slice/1(I) -> " I"/1
  I/Q Concat/1(IQ) -> FIFO/1
  Write/1 -> FIFO/2
  [TX_RESET] -> Delay1/1
  FIFO/1 -> I/Q Slice/1(IQ)
  FIFO/4 -> " Occ"/1
  Rd/1 -> FIFO/3
  Delay1/1 -> Logical4/1
  Reset/1 -> Convert2/1
  Logical4/1 -> FIFO/4
  Convert2/1 -> Logical4/2

== system wlan_phy_tx_pmd/Preamble & Outputs/Posedge ==
  D : Inport
  Delay : xbsIndex_r4/Delay  rst=off  infoeditControl=Selection of Reset will increase slice count due to use of real FFs and instead of SRLs  en=off  latency=1  dbl_ovrd=off  reg_retiming=off  block_type=delay
      settings: infoedit=Hardware notes: A delay line is a chain, each link of which is an SRL16 followed by a flip-flop. If register retiming is enabled, the delay line is a chain of flip-flops.  xl_area=[1 1 0 0 0 0 0]  block_version=VER_STRING_GOES_HERE
  Inverter : xbsIndex_r4/Inverter  en=off  latency=0  dbl_ovrd=off  block_type=inv
      settings: xl_area=[0 0 0 0 0 0 0]  block_version=VER_STRING_GOES_HERE
  Logical1 : xbsIndex_r4/Logical  logical_function=AND  inputs=2  en=off  latency=0  precision=Full  arith_type=Unsigned  n_bits=8  bin_pt=2  align_bp=on  dbl_ovrd=off  block_type=logical
      settings: xl_area=[1 0 0 1 0 0 0]  block_version=VER_STRING_GOES_HERE
  Q : Outport
  wires:
  D/1 -> Logical1/2, Delay/1
  Logical1/1 -> Q/1
  Inverter/1 -> Logical1/1
  Delay/1 -> Inverter/1

== system wlan_phy_tx_pmd/Preamble & Outputs/Preamble Gen ==
  note: Synchronize preamble samples to the read_en signal
      | so the inputs to the mux are aligned
  note: TX_RESET asserts at the end of each Tx.
      | Delay it here to give the FIFO/MUX latencies
      | time to flush the last few samples before switching
      | the mux back to the preamble, for the next Tx.
  Tx Running : Inport
  Rd En : Inport  Port=2
  Constant3 : xbsIndex_r4/Constant  const=length(Preamble_IQ)-1  gui_display_data_type=Fixed-point  arith_type=Unsigned  n_bits=ceil(log2(length(Preamble_IQ)))  bin_pt=0  preci_type=Single  exp_width=8  frac_width=24  explicit_period=off  period=1  equ=P=C  opselect=C  inp2=PCIN>>17  opr=+  inp1=P  carry=CIN  dbl_ovrd=off  block_type=constant
  Counter : xbsIndex_r4/Counter  cnt_type=Free Running  cnt_to=Inf  operation=Up  start_count=0  cnt_by_val=1  arith_type=Unsigned  n_bits=ceil(log2(length(Preamble_IQ)))  bin_pt=0  load_pin=off  rst=on  en=on  explicit_period=off  period=1  dbl_ovrd=off  use_behavioral_HDL=off  implementation=Fabric  block_type=counter
  Delay4 : xbsIndex_r4/Delay  rst=off  infoeditControl=Selection of Reset will increase slice count due to use of real FFs and instead of SRLs  en=off  latency=4  dbl_ovrd=off  reg_retiming=off  block_type=delay
  Inverter1 : xbsIndex_r4/Inverter  en=off  latency=0  dbl_ovrd=off  block_type=inv
      settings: xl_area=[0 0 0 0 0 0 0]  block_version=VER_STRING_GOES_HERE
  Logical1 : xbsIndex_r4/Logical  logical_function=AND  inputs=3  en=off  latency=0  precision=Full  arith_type=Unsigned  n_bits=16  bin_pt=0  align_bp=on  dbl_ovrd=off  block_type=logical
  Preamble I : xbsIndex_r4/ROM  depth=length(Preamble_IQ_scaled)  initVector=real(Preamble_IQ_scaled)  distributed_mem=Distributed memory  rst=off  init_reg=0  en=off  latency=1  gui_display_data_type=Fixed-point  arith_type="Signed  (2's comp)"  n_bits=16  bin_pt=15  preci_type=Single  exp_width=8  frac_width=24  dbl_ovrd=off  optimize=Area  use_rpm=on  block_type=sprom
  Preamble Q : xbsIndex_r4/ROM  depth=length(Preamble_IQ_scaled)  initVector=imag(Preamble_IQ_scaled)  distributed_mem=Distributed memory  rst=off  init_reg=0  en=off  latency=1  gui_display_data_type=Fixed-point  arith_type="Signed  (2's comp)"  n_bits=16  bin_pt=15  preci_type=Single  exp_width=8  frac_width=24  dbl_ovrd=off  optimize=Area  use_rpm=on  block_type=sprom
  Register{,1..3} (4 alike) : xbsIndex_r4/Register  init=0  rst=on  en=on  dbl_ovrd=off  block_type=register
  Relational2 : xbsIndex_r4/Relational  mode=a<b  en=off  latency=0  dbl_ovrd=off  block_type=relational
  Done : Outport
  I : Outport  Port=2
  Q : Outport  Port=3
  Early Done : Outport  Port=4
  wires:
  Counter/1 -> Preamble I/1, Preamble Q/1, Relational2/1
  [TX_RESET] -> Delay4/1
  Logical1/1 -> Counter/2
  Relational2/1 -> Logical1/3, Inverter1/1
  Constant3/1 -> Relational2/2
  Tx Running/1 -> Logical1/1
  Rd En/1 -> Logical1/2, Register1/3, Register2/3, Register3/3, Register/3
  Preamble I/1 -> Register2/1
  Preamble Q/1 -> Register3/1
  Register/1 -> Early Done/1, Register1/1
  Delay4/1 -> Counter/1, Register/2, Register1/2, Register2/2, Register3/2
  Inverter1/1 -> Register/1
  Register1/1 -> Done/1
  Register2/1 -> I/1
  Register3/1 -> Q/1

== system wlan_phy_tx_pmd/Preamble & Outputs/S-R Latch ==
  S : Inport
  R : Inport  Port=2
  Constant1 : xbsIndex_r4/Constant  const=1  gui_display_data_type=Fixed-point  arith_type=Boolean  n_bits=1  bin_pt=0  preci_type=Single  exp_width=8  frac_width=24  explicit_period=off  period=1  equ=P=C  opselect=C  inp2=PCIN>>17  opr=+  inp1=P  carry=CIN  dbl_ovrd=off  block_type=constant
      settings: block_version=VER_STRING_GOES_HERE
  Convert1 : xbsIndex_r4/Convert  gui_display_data_type=Boolean  arith_type=Boolean  n_bits=1  bin_pt=0  float_type=Single  exp_bits=8  fraction_bits=24  quantization=Truncate  overflow=Wrap  en=off  latency=0  dbl_ovrd=off  pipeline=off  block_type=convert
  Convert2 : xbsIndex_r4/Convert  gui_display_data_type=Boolean  arith_type=Boolean  n_bits=1  bin_pt=0  float_type=Single  exp_bits=8  fraction_bits=24  quantization=Truncate  overflow=Wrap  en=off  latency=0  dbl_ovrd=off  pipeline=off  block_type=convert
  Register2 : xbsIndex_r4/Register  init=0  rst=on  en=on  dbl_ovrd=off  block_type=register
      settings: xl_area=[1 1 0 0 0 0 0]  block_version=VER_STRING_GOES_HERE
  Q : Outport
  wires:
  Convert2/1 -> Register2/3
  Convert1/1 -> Register2/2
  Constant1/1 -> Register2/1
  R/1 -> Convert1/1
  Register2/1 -> Q/1
  S/1 -> Convert2/1

== system wlan_phy_tx_pmd/Preamble & Outputs/S-R Latch1 ==
  S : Inport
  R : Inport  Port=2
  Constant1 : xbsIndex_r4/Constant  const=1  gui_display_data_type=Fixed-point  arith_type=Boolean  n_bits=1  bin_pt=0  preci_type=Single  exp_width=8  frac_width=24  explicit_period=off  period=1  equ=P=C  opselect=C  inp2=PCIN>>17  opr=+  inp1=P  carry=CIN  dbl_ovrd=off  block_type=constant
      settings: block_version=VER_STRING_GOES_HERE
  Convert1 : xbsIndex_r4/Convert  gui_display_data_type=Boolean  arith_type=Boolean  n_bits=1  bin_pt=0  float_type=Single  exp_bits=8  fraction_bits=24  quantization=Truncate  overflow=Wrap  en=off  latency=0  dbl_ovrd=off  pipeline=off  block_type=convert
  Convert2 : xbsIndex_r4/Convert  gui_display_data_type=Boolean  arith_type=Boolean  n_bits=1  bin_pt=0  float_type=Single  exp_bits=8  fraction_bits=24  quantization=Truncate  overflow=Wrap  en=off  latency=0  dbl_ovrd=off  pipeline=off  block_type=convert
  Register2 : xbsIndex_r4/Register  init=0  rst=on  en=on  dbl_ovrd=off  block_type=register
      settings: xl_area=[1 1 0 0 0 0 0]  block_version=VER_STRING_GOES_HERE
  Q : Outport
  wires:
  S/1 -> Convert2/1
  Register2/1 -> Q/1
  R/1 -> Convert1/1
  Constant1/1 -> Register2/1
  Convert1/1 -> Register2/2
  Convert2/1 -> Register2/3

== system wlan_phy_tx_pmd/Preamble & Outputs/Scaling ==
  Preamble : Inport
  I : Inport  Port=2
  Q : Inport  Port=3
  Display : Display
  Display1 : Display
  Gateway Out1 : xbsIndex_r4/Gateway Out  inherit_from_input=off  hdl_port=off  timing_constraint=None  locs_specified=off  LOCs={}  UseAsDAC=off  DACChannel='1'  block_type=gatewayout
  Gateway Out5 : xbsIndex_r4/Gateway Out  inherit_from_input=off  hdl_port=off  timing_constraint=None  locs_specified=off  LOCs={}  UseAsDAC=off  DACChannel='1'  block_type=gatewayout
  Mult : xbsIndex_r4/Mult  precision=User Defined  arith_type="Signed  (2's comp)"  n_bits=12  bin_pt=11  quantization=Truncate  overflow=Saturate  en=off  latency=1  dbl_ovrd=off  use_behavioral_HDL=off  opt=Speed  use_embedded=on  optimum_pipeline=off  pipeline=on  use_rpm=on  placement_style=Triangular  block_type=mult
  Mult1 : xbsIndex_r4/Mult  precision=User Defined  arith_type="Signed  (2's comp)"  n_bits=12  bin_pt=11  quantization=Truncate  overflow=Saturate  en=off  latency=1  dbl_ovrd=off  use_behavioral_HDL=off  opt=Speed  use_embedded=on  optimum_pipeline=off  pipeline=on  use_rpm=on  placement_style=Triangular  block_type=mult
  Mux1 : xbsIndex_r4/Mux  inputs=2  en=off  latency=0  precision=Full  arith_type=Unsigned  n_bits=16  bin_pt=14  quantization=Truncate  overflow=Wrap  dbl_ovrd=off  block_type=mux
  " I" : Outport
  " Q" : Outport  Port=2
  wires:
  Mult/1 -> " I"/1
  Mult1/1 -> " Q"/1
  I/1 -> Mult/1
  Q/1 -> Mult1/2
  Mux1/1 -> Mult/2, Mult1/1
  [regTx_Scaling_Payload] -> Mux1/2, Gateway Out5/1
  Preamble/1 -> Mux1/1
  [regTx_Scaling_Preamble] -> Mux1/3, Gateway Out1/1
  Gateway Out5/1 -> Display/1
  Gateway Out1/1 -> Display1/1

== system wlan_phy_tx_pmd/Registers/Status Bits ==
  Concat : xbsIndex_r4/Concat  num_inputs=2  dbl_ovrd=off  block_type=concat
  Constant : xbsIndex_r4/Constant  const=0  gui_display_data_type=Fixed-point  arith_type=Unsigned  n_bits=31  bin_pt=0  preci_type=Single  exp_width=8  frac_width=24  explicit_period=off  period=1  equ=P=C  opselect=C  inp2=PCIN>>17  opr=+  inp1=P  carry=CIN  dbl_ovrd=off  block_type=constant
  32b : Outport
  wires:
  [regTx_TX_RUNNING] -> Concat/2
  Constant/1 -> Concat/1
  Concat/1 -> 32b/1

== system wlan_phy_tx_pmd/Resets/Posedge1 ==
  note: Rising Edge Detection
  D : Inport
  Delay : xbsIndex_r4/Delay  rst=off  infoeditControl=Selection of Reset will increase slice count due to use of real FFs and instead of SRLs  en=off  latency=1  dbl_ovrd=off  reg_retiming=off  block_type=delay
      settings: infoedit=Hardware notes: A delay line is a chain, each link of which is an SRL16 followed by a flip-flop. If register retiming is enabled, the delay line is a chain of flip-flops.  xl_area=[1 1 0 0 0 0 0]  block_version=VER_STRING_GOES_HERE
  Inverter : xbsIndex_r4/Inverter  en=off  latency=0  dbl_ovrd=off  block_type=inv
      settings: xl_area=[0 0 0 0 0 0 0]  block_version=VER_STRING_GOES_HERE
  Logical1 : xbsIndex_r4/Logical  logical_function=AND  inputs=2  en=off  latency=0  precision=Full  arith_type=Unsigned  n_bits=8  bin_pt=2  align_bp=on  dbl_ovrd=off  block_type=logical
      settings: xl_area=[1 0 0 1 0 0 0]  block_version=VER_STRING_GOES_HERE
  Q : Outport
  wires:
  Delay/1 -> Inverter/1
  Inverter/1 -> Logical1/1
  Logical1/1 -> Q/1
  D/1 -> Delay/1, Logical1/2
